simulink library "myLibrary"  (R2023b)
settings: Solver=VariableStepAuto  StartTime=0.0  StopTime=10.0  RelTol=1e-3
undefined symbols (not defined in the file): Cac_n1, ctrl1, Da, Discrete, dtha, ee_sli_rtmsupport, FA, gcbh, Ha, Ini, init_DCline, init_IPC, init_line, init_load, init_SG, init_shunt, init_TH, init_trafo, init_VSC, initMachineBlocks, Ka, Lf, Llkd_pu, Llkq1_pu, magnitude, NET, P, plots_step, q0, Rac_n1, Radd, Rkd_pu, Rkq1_pu, Rload_add, sim_config, sps_rtmsupport, spsSteamTurbineModel, T_DC_NET, T_global, T_IPC, T_load, T_NET, T_SG, T_shunt, T_STATCOM, T_TH, T_trafo, T_VSC, Ts, tstep, Udiff_a, V1
libraries: spsSeriesRLCBranchLib x105, eeGeneralControl x72, $bdroot x70, spsCurrentMeasurementLib x48, spsParallelRLCBranchLib x39, spsVoltageMeasurementLib x33, spsControlledVoltageSourceLib x27, spsFirstOrderFilterLib x16, dspsigops x6, spsThreePhaseVIMeasurementLib x5, spsPLL3phLib x4, spsThreePhaseBreakerLib x3
(part 7 of 12)

== system myLibrary/AC-GFOL_DC-GFOL/Control Pac2/PLL1 ==
  Ud : Inport
  Constant : Constant  Value=0
  Constant1 : Constant  Value=2*pi*T_IPC.fb
  Gain : Gain  Gain=T_IPC.kiPLL
  Gain1 : Gain  Gain=T_IPC.kpPLL
  Integrator : Integrator  InitialCondition=initIPC.thetaPLL_init
  Integrator1 : Integrator
  Scope : Scope
  Scope1 : Scope  NumInputPorts=2
  Sum : Sum  Inputs=|+-
  Sum1 : Sum  Inputs=|++
  Sum2 : Sum  Inputs=|++
  Angle : Outport
  w : Outport  Port=2
  wires:
  Ud/1 -> Scope1/2, Sum/2
  Constant1/1 -> Sum2/2
  Sum2/1 -> w/1, Scope/1, Integrator/1
  Sum1/1 -> Sum2/1
  Integrator1/1 -> Sum1/2
  Gain1/1 -> Sum1/1
  Gain/1 -> Integrator1/1
  Sum/1 -> Gain1/1, Gain/1
  Constant/1 -> Scope1/1, Sum/1
  Integrator/1 -> Angle/1

== system myLibrary/AC-GFOL_DC-GFOL/Control Pac2/Rotació ==
  V_q_diff : Inport
  V_d_diff : Inport  Port=2
  V_0_diff : Inport  Port=3
  Angle : Inport  Port=4
  Constant{2,5..7} (4 alike) : Constant  Value=0
  Constant8 : Constant
  Demux : Demux  Outputs=3
  Display : Display
  Gain1 : Gain  Gain=-1
  Matrix Concatenate : Concatenate  NumInputs=3  Mode=Multidimensional array  ConcatenateDimension=2
  Mux{,1..3} (4 alike) : Mux  Inputs=3
  Product : Product  Multiplication=Matrix(*)
  Trigonometric Function : Trigonometry  Operator=cos
  Trigonometric Function1 : Trigonometry
  Trigonometric Function2 : Trigonometry
  Trigonometric Function3 : Trigonometry  Operator=cos
  V_alfa_diff : Outport  VectorParamsAs1DForOutWhenUnconnected=off
  V_beta_diff : Outport  Port=2  VectorParamsAs1DForOutWhenUnconnected=off
  V_0 : Outport  Port=3  VectorParamsAs1DForOutWhenUnconnected=off
  wires:
  Trigonometric Function1/1 -> Gain1/1
  Constant2/1 -> Mux1/3
  Trigonometric Function3/1 -> Mux2/2
  Constant5/1 -> Mux2/3
  Constant6/1 -> Mux3/1
  Constant7/1 -> Mux3/2
  Constant8/1 -> Mux3/3
  Mux2/1 -> Matrix Concatenate/2
  Mux3/1 -> Matrix Concatenate/3
  Mux1/1 -> Matrix Concatenate/1
  Product/1 -> Demux/1
  Demux/1 -> V_alfa_diff/1
  Demux/2 -> V_beta_diff/1
  Demux/3 -> V_0/1
  Mux/1 -> Product/2
  Matrix Concatenate/1 -> Display/1, Product/1
  V_q_diff/1 -> Mux/1
  V_d_diff/1 -> Mux/2
  V_0_diff/1 -> Mux/3
  Trigonometric Function/1 -> Mux1/1
  Gain1/1 -> Mux1/2
  Trigonometric Function2/1 -> Mux2/1
  Angle/1 -> Trigonometric Function/1, Trigonometric Function3/1, Trigonometric Function2/1, Trigonometric Function1/1

== system myLibrary/AC-GFOL_DC-GFOL/Control Pac2/Subsystem ==
  iqs : Inport
  uq : Inport  Port=2
  ids : Inport  Port=3
  ud : Inport  Port=4
  w : Inport  Port=5
  Pac_ref : Inport  Port=6
  Constant : Constant  Value=T_IPC.fb*2*pi
  Display5 : Display
  Gain1 : Gain  Gain=T_IPC.kpw
  Gain2 : Gain  Gain=3/2
  Integrator1 : Integrator  InitialCondition=initIPC.idiffq
  Product3 : Product
  Product5 : Product
  Scope : Scope  NumInputPorts=2
  Scope1 : Scope
  Sum1 : Sum
  Sum10 : Sum  Inputs=|++
  Sum2 : Sum  Inputs=++-
  Sum3 : Sum  Inputs=|+-
  k7 : Gain  Gain=T_IPC.kiPac
  k8 : Gain  Gain=T_IPC.kpPac
  iqref : Outport
  wires:
  Constant/1 -> Sum3/1
  w/1 -> Sum3/2
  Sum3/1 -> Gain1/1
  Gain2/1 -> Sum2/3, Scope/2  "V_0_"
  iqs/1 -> Product3/2
  Product5/1 -> Sum1/2
  uq/1 -> Product3/1
  ids/1 -> Product5/2
  Sum1/1 -> Gain2/1  "V_0_s"
  ud/1 -> Product5/1
  Product3/1 -> Sum1/1
  Pac_ref/1 -> Scope/1, Sum2/2
  Integrator1/1 -> Display5/1, Scope1/1, Sum10/2
  k7/1 -> Integrator1/1
  k8/1 -> Sum10/1
  Sum2/1 -> k7/1, k8/1
  Sum10/1 -> iqref/1

== system myLibrary/AC-GFOL_DC-GFOL/Control Pac2/Subsystem1 ==
  uref : Inport
  uq : Inport  Port=2
  ud : Inport  Port=3
  Gain3 : Gain  Gain=T_IPC.kpVac
  Low-Pass Filter (Discrete or Continuous)2 : eeGeneralControl/Low-Pass Filter (Discrete or Continuous)  K=1  T=T_IPC.tVac  B=inf  A=-inf  init_option=Inherited from block input  x0=0  Ts=0
  Product4 : Product
  Product6 : Product
  Scope : Scope  NumInputPorts=2
  Sqrt : Sqrt
  Sum : Sum
  Sum3 : Sum  Inputs=|+-
  idref : Outport
  wires:
  uref/1 -> Scope/1, Sum3/1
  Product6/1 -> Sum/2
  Sqrt/1 -> Low-Pass Filter (Discrete or Continuous)2/1, Scope/2
  uq/1 -> Product4/2, Product4/1
  Sum/1 -> Sqrt/1
  ud/1 -> Product6/2, Product6/1
  Gain3/1 -> idref/1  "V_0_"
  Product4/1 -> Sum/1
  Low-Pass Filter (Discrete or Continuous)2/1 -> Sum3/2
  Sum3/1 -> Gain3/1

== system myLibrary/AC-GFOL_DC-GFOL/Control Pac2/Subsystem2 ==
  iqs : Inport
  uq : Inport  Port=2
  ids : Inport  Port=3
  ud : Inport  Port=4
  Pac_ref : Inport  Port=5
  Display5 : Display
  Gain2 : Gain  Gain=3/2
  Integrator1 : Integrator  InitialCondition=initIPC.idiffd
  Product3 : Product
  Product5 : Product
  Scope : Scope  NumInputPorts=2
  Scope1 : Scope
  Sum1 : Sum  Inputs=+-
  Sum10 : Sum  Inputs=|++
  Sum2 : Sum  Inputs=|+-
  k7 : Gain  Gain=T_IPC.kiQ
  k8 : Gain  Gain=T_IPC.kpQ
  iqref : Outport
  wires:
  Sum10/1 -> iqref/1
  Sum2/1 -> k8/1, k7/1
  k8/1 -> Sum10/1
  k7/1 -> Integrator1/1
  Integrator1/1 -> Scope1/1, Sum10/2, Display5/1
  Pac_ref/1 -> Sum2/1, Scope/1
  Product3/1 -> Sum1/1
  ud/1 -> Product5/1
  Sum1/1 -> Gain2/1  "V_0_s"
  uq/1 -> Product3/1
  Product5/1 -> Sum1/2
  Gain2/1 -> Sum2/2, Scope/2  "V_0_"
  ids/1 -> Product3/2
  iqs/1 -> Product5/2

== system myLibrary/AC-GFOL_DC-GFOL/Control Pac2/l_DC_alfa//beta ==
  Iabc_sum : Inport
  Clarke : Subsystem
  Ialfa_sum : Outport  VectorParamsAs1DForOutWhenUnconnected=off
  Ibeta_sum : Outport  Port=2  VectorParamsAs1DForOutWhenUnconnected=off
  I0_sum : Outport  Port=3  VectorParamsAs1DForOutWhenUnconnected=off
  wires:
  Clarke/1(I_alfa) -> Ialfa_sum/1
  Clarke/2(I_beta) -> Ibeta_sum/1
  Clarke/3(I_0) -> I0_sum/1
  Iabc_sum/1 -> Clarke/1(Isum)

== system myLibrary/AC-GFOL_DC-GFOR/Control Pac2/Calcul Energies2 ==
  Vs : Inport
  Demux : Demux  Outputs=6
  Gain{1..6} (6 alike) : Gain  Gain=T_IPC.Carm/2
  Math Function{1..6} (6 alike) : Math  Operator=magnitude^2  SignedPower=on
  Sum4 : Sum  Inputs=|++
  Sum5 : Sum  Inputs=|++
  Sum9 : Sum  Inputs=|++
  Eat : Outport
  Ebt : Outport  Port=2
  Ect : Outport  Port=3
  wires:
  [Ebl] -> Sum5/2
  Gain5/1 -> [Ecu]  "Ecu"
  [Eau] -> Sum4/1
  Gain1/1 -> [Eau]  "Eau"
  Gain2/1 -> [Eal]  "Eal"
  [Ecu] -> Sum9/1
  Math Function4/1 -> Gain4/1
  [Ecl] -> Sum9/2
  Math Function1/1 -> Gain1/1
  Gain4/1 -> [Ebl]  "Ebl"
  [Ebu] -> Sum5/1
  Gain6/1 -> [Ecl]  "Ecl"
  Sum9/1 -> Ect/1
  Math Function5/1 -> Gain5/1
  [Vcls] -> Math Function6/1
  Math Function2/1 -> Gain2/1
  [Vbus] -> Math Function3/1
  Sum5/1 -> Ebt/1
  Math Function6/1 -> Gain6/1
  [Vals] -> Math Function2/1
  [Vaus] -> Math Function1/1
  Math Function3/1 -> Gain3/1
  Sum4/1 -> Eat/1
  Gain3/1 -> [Ebu]  "Ebu"
  [Eal] -> Sum4/2
  [Vcus] -> Math Function5/1
  [Vbls] -> Math Function4/1
  Vs/1 -> Demux/1
  Demux/1 -> [Vaus]
  Demux/2 -> [Vals]
  Demux/3 -> [Vbus]
  Demux/4 -> [Vbls]
  Demux/5 -> [Vcus]
  Demux/6 -> [Vcls]

== system myLibrary/AC-GFOL_DC-GFOR/Control Pac2/Clarke Anti-Transformation ==
  V_alfa_diff : Inport
  V_beta_dfff : Inport  Port=2
  V_0_diff : Inport  Port=3
  Constant{,2,5,8} (4 alike) : Constant
  Constant1 : Constant  Value=0
  Constant3 : Constant  Value=-1/2
  Constant4 : Constant  Value=-sqrt(3)/2
  Constant6 : Constant  Value=-1/2
  Constant7 : Constant  Value=sqrt(3)/2
  Demux : Demux  Outputs=3
  Display : Display
  Math Function : Math  Operator=transpose  SignedPower=on
  Matrix Concatenate : Concatenate  NumInputs=3  Mode=Multidimensional array  ConcatenateDimension=2
  Mux{,1..3} (4 alike) : Mux  Inputs=3
  Product : Product  Multiplication=Matrix(*)
  Va_diff : Outport  VectorParamsAs1DForOutWhenUnconnected=off
  Vb_diff : Outport  Port=2  VectorParamsAs1DForOutWhenUnconnected=off
  Vc_diff : Outport  Port=3  VectorParamsAs1DForOutWhenUnconnected=off
  wires:
  Constant/1 -> Mux1/1
  Constant1/1 -> Mux1/2
  Constant2/1 -> Mux1/3
  Constant3/1 -> Mux2/1
  Constant4/1 -> Mux2/2
  Constant5/1 -> Mux2/3
  Constant6/1 -> Mux3/1
  Constant7/1 -> Mux3/2
  Constant8/1 -> Mux3/3
  Matrix Concatenate/1 -> Math Function/1
  Mux2/1 -> Matrix Concatenate/2
  Mux3/1 -> Matrix Concatenate/3
  Mux1/1 -> Matrix Concatenate/1
  Product/1 -> Demux/1
  Demux/1 -> Va_diff/1  "Va"
  Demux/2 -> Vb_diff/1  "Vb"
  Demux/3 -> Vc_diff/1  "Vc"
  Mux/1 -> Product/2
  Math Function/1 -> Display/1, Product/1
  V_alfa_diff/1 -> Mux/1  "Valfa"
  V_beta_dfff/1 -> Mux/2  "Vbeta"
  V_0_diff/1 -> Mux/3  "0"

== system myLibrary/AC-GFOL_DC-GFOR/Control Pac2/Clarke Anti-Transformation2 ==
  V_alfa_sum : Inport
  V_beta_sum : Inport  Port=2
  V_0_sum : Inport  Port=3
  Constant{,2,5,8} (4 alike) : Constant
  Constant1 : Constant  Value=0
  Constant3 : Constant  Value=-1/2
  Constant4 : Constant  Value=-sqrt(3)/2
  Constant6 : Constant  Value=-1/2
  Constant7 : Constant  Value=sqrt(3)/2
  Demux : Demux  Outputs=3
  Display : Display
  Math Function : Math  Operator=transpose  SignedPower=on
  Matrix Concatenate : Concatenate  NumInputs=3  Mode=Multidimensional array  ConcatenateDimension=2
  Mux{,1..3} (4 alike) : Mux  Inputs=3
  Product : Product  Multiplication=Matrix(*)
  Va_sum : Outport  VectorParamsAs1DForOutWhenUnconnected=off
  Vb_sum : Outport  Port=2  VectorParamsAs1DForOutWhenUnconnected=off
  Vc_sum : Outport  Port=3  VectorParamsAs1DForOutWhenUnconnected=off
  wires:
  Constant/1 -> Mux1/1
  Constant1/1 -> Mux1/2
  Constant2/1 -> Mux1/3
  Constant3/1 -> Mux2/1
  Constant4/1 -> Mux2/2
  Constant5/1 -> Mux2/3
  Constant6/1 -> Mux3/1
  Constant7/1 -> Mux3/2
  Constant8/1 -> Mux3/3
  Matrix Concatenate/1 -> Math Function/1
  Mux2/1 -> Matrix Concatenate/2
  Mux3/1 -> Matrix Concatenate/3
  Mux1/1 -> Matrix Concatenate/1
  Product/1 -> Demux/1
  Demux/1 -> Va_sum/1  "Va"
  Demux/2 -> Vb_sum/1  "Vb"
  Demux/3 -> Vc_sum/1  "Vc"
  Mux/1 -> Product/2
  Math Function/1 -> Display/1, Product/1
  V_alfa_sum/1 -> Mux/1  "Valfa"
  V_beta_sum/1 -> Mux/2  "Vbeta"
  V_0_sum/1 -> Mux/3  "0"

== system myLibrary/AC-GFOL_DC-GFOR/Control Pac2/Conditional zoh1 ==
  In1 : Inport
  Constant4 : Constant  Value=T_IPC.tau_zoh
  Switch : Switch  Criteria=u2 > Threshold  SaturateOnIntegerOverflow=off  InputSameDT=off
  Zero-Order Hold9 : ZeroOrderHold  SampleTime=T_IPC.tau_zoh
  Out1 : Outport
  wires:
  In1/1 -> Zero-Order Hold9/1, Switch/3
  Zero-Order Hold9/1 -> Switch/1
  Constant4/1 -> Switch/2
  Switch/1 -> Out1/1

== system myLibrary/AC-GFOL_DC-GFOR/Control Pac2/Conditional zoh5 ==
  In1 : Inport
  Constant4 : Constant  Value=T_IPC.tau_zoh
  Switch : Switch  Criteria=u2 > Threshold  SaturateOnIntegerOverflow=off  InputSameDT=off
  Zero-Order Hold9 : ZeroOrderHold  SampleTime=T_IPC.tau_zoh
  Out1 : Outport
  wires:
  In1/1 -> Zero-Order Hold9/1, Switch/3
  Zero-Order Hold9/1 -> Switch/1
  Constant4/1 -> Switch/2
  Switch/1 -> Out1/1

== system myLibrary/AC-GFOL_DC-GFOR/Control Pac2/Conditional zoh7 ==
  In1 : Inport
  Constant4 : Constant  Value=T_IPC.tau_zoh
  Switch : Switch  Criteria=u2 > Threshold  SaturateOnIntegerOverflow=off  InputSameDT=off
  Zero-Order Hold9 : ZeroOrderHold  SampleTime=T_IPC.tau_zoh
  Out1 : Outport
  wires:
  Switch/1 -> Out1/1
  Constant4/1 -> Switch/2
  Zero-Order Hold9/1 -> Switch/1
  In1/1 -> Switch/3, Zero-Order Hold9/1

== system myLibrary/AC-GFOL_DC-GFOR/Control Pac2/Conditional zoh8 ==
  In1 : Inport
  Constant4 : Constant  Value=T_IPC.tau_zoh
  Switch : Switch  Criteria=u2 > Threshold  SaturateOnIntegerOverflow=off  InputSameDT=off
  Zero-Order Hold9 : ZeroOrderHold  SampleTime=T_IPC.tau_zoh
  Out1 : Outport
  wires:
  Switch/1 -> Out1/1
  Constant4/1 -> Switch/2
  Zero-Order Hold9/1 -> Switch/1
  In1/1 -> Switch/3, Zero-Order Hold9/1

== system myLibrary/AC-GFOL_DC-GFOR/Control Pac2/Control Energies DC ==
  Pt : Inport
  Display1 : Display
  Integrator1 : Integrator  InitialCondition=initIPC.PI_Wt
  Scope : Scope
  Sum10 : Sum  Inputs=|++
  k7 : Gain  Gain=T_IPC.kiEt
  k8 : Gain  Gain=T_IPC.kpEt
  Pt' : Outport  VectorParamsAs1DForOutWhenUnconnected=off
  wires:
  Sum10/1 -> Pt'/1  "Pt"
  k7/1 -> Integrator1/1
  Pt/1 -> k7/1, k8/1
  k8/1 -> Sum10/1
  Integrator1/1 -> Scope/1, Sum10/2, Display1/1

== system myLibrary/AC-GFOL_DC-GFOR/Control Pac2/Controladors ==
  I_0_sum : Inport
  Display : Display
  Gain2 : Gain  Gain=-1
  Integrator1 : Integrator  InitialCondition=initIPC.PI_isum0_DC
  Ki1 : Gain  Gain=T_IPC.kiIsum
  Kp1 : Gain  Gain=T_IPC.kpIsum
  Scope : Scope
  Sum5 : Sum
  V_0_sum : Outport  VectorParamsAs1DForOutWhenUnconnected=off
  wires:
  Sum5/1 -> Gain2/1
  Gain2/1 -> V_0_sum/1
  Ki1/1 -> Integrator1/1
  Integrator1/1 -> Display/1, Scope/1, Sum5/1
  Kp1/1 -> Sum5/2
  I_0_sum/1 -> Kp1/1, Ki1/1

== system myLibrary/AC-GFOL_DC-GFOR/Control Pac2/Current Control ==
  Iq* : Inport
  Iq : Inport  Port=2
  Id* : Inport  Port=3
  Id : Inport  Port=4
  uq : Inport  Port=5
  ud : Inport  Port=6
  Constant : Constant  Value=2*pi*T_IPC.fb
  Display1 : Display
  Display6 : Display
  Id1 : InportShadow  Port=4
  Integrator : Integrator  InitialCondition=initIPC.PI_idiffq
  Integrator1 : Integrator  InitialCondition=initIPC.PI_idiffd
  Iq1 : InportShadow  Port=2
  Ki : Gain  Gain=T_IPC.kiIs
  Ki1 : Gain  Gain=T_IPC.kiIs
  Kp : Gain  Gain=T_IPC.kpIs
  Kp1 : Gain  Gain=T_IPC.kpIs
  Kp2 : Gain  Gain=T_IPC.Lc+T_IPC.La/2
  Product : Product
  Product1 : Product
  Scope : Scope  NumInputPorts=2
  Scope1 : Scope  NumInputPorts=2
  Sum : Sum  Inputs=|+-
  Sum1 : Sum  Inputs=|+-
  Sum2 : Sum  Inputs=+++
  Sum3 : Sum  Inputs=-++
  Sum4 : Sum
  Sum5 : Sum
  V_q_s : Outport  VectorParamsAs1DForOutWhenUnconnected=off
  V_d_s : Outport  Port=2  VectorParamsAs1DForOutWhenUnconnected=off
  wires:
  Sum2/1 -> V_q_s/1
  Sum5/1 -> Sum3/2
  Kp1/1 -> Sum5/2
  Integrator1/1 -> Display1/1, Sum5/1
  Ki1/1 -> Integrator1/1
  Sum1/1 -> Ki1/1, Kp1/1  "Error"
  Kp/1 -> Sum4/2
  Integrator/1 -> Display6/1, Sum4/1
  Ki/1 -> Integrator/1
  Sum/1 -> Kp/1, Ki/1
  Id*/1 -> Scope1/1, Sum1/1
  Kp2/1 -> Product/2, Product1/1
  Id/1 -> Scope1/2, Sum1/2
  Iq/1 -> Scope/2, Sum/2
  Iq*/1 -> Scope/1, Sum/1
  Constant/1 -> Kp2/1
  ud/1 -> Sum3/3
  Sum4/1 -> Sum2/1
  uq/1 -> Sum2/3
  Sum3/1 -> V_d_s/1
  Product/1 -> Sum3/1
  Product1/1 -> Sum2/2
  Iq1/1 -> Product/1
  Id1/1 -> Product1/2

== system myLibrary/AC-GFOL_DC-GFOR/Control Pac2/Is ==
  Ias : Inport
  Ibs : Inport  Port=2
  Ics : Inport  Port=3
  Angle : Inport  Port=4
  Demux1 : Demux  Outputs=3
  Matriu T : Subsystem
  Mux : Mux  Inputs=3
  Product : Product  Multiplication=Matrix(*)
  I_q_s : Outport  VectorParamsAs1DForOutWhenUnconnected=off
  I_d_s : Outport  Port=2  VectorParamsAs1DForOutWhenUnconnected=off
  I_0_s : Outport  Port=3  VectorParamsAs1DForOutWhenUnconnected=off
  wires:
  Product/1 -> Demux1/1
  Matriu T/1(Out1) -> Product/1
  Demux1/1 -> I_q_s/1
  Demux1/2 -> I_d_s/1
  Demux1/3 -> I_0_s/1
  Angle/1 -> Matriu T/1(u)
  Mux/1 -> Product/2
  Ias/1 -> Mux/1
  Ibs/1 -> Mux/2
  Ics/1 -> Mux/3

== system myLibrary/AC-GFOL_DC-GFOR/Control Pac2/Is2 ==
  Ias : Inport
  Ibs : Inport  Port=2
  Ics : Inport  Port=3
  Angle : Inport  Port=4
  Demux1 : Demux  Outputs=3
  Matriu T : Subsystem
  Mux : Mux  Inputs=3
  Product : Product  Multiplication=Matrix(*)
  I_q_s : Outport  VectorParamsAs1DForOutWhenUnconnected=off
  I_d_s : Outport  Port=2  VectorParamsAs1DForOutWhenUnconnected=off
  I_0_s : Outport  Port=3  VectorParamsAs1DForOutWhenUnconnected=off
  wires:
  Product/1 -> Demux1/1
  Matriu T/1(Out1) -> Product/1
  Demux1/1 -> I_q_s/1
  Demux1/2 -> I_d_s/1
  Demux1/3 -> I_0_s/1
  Angle/1 -> Matriu T/1(u)
  Mux/1 -> Product/2
  Ias/1 -> Mux/1
  Ibs/1 -> Mux/2
  Ics/1 -> Mux/3

== system myLibrary/AC-GFOL_DC-GFOR/Control Pac2/PLL1 ==
  Ud : Inport
  Constant : Constant  Value=0
  Constant1 : Constant  Value=2*pi*T_IPC.fb
  Gain : Gain  Gain=T_IPC.kiPLL
  Gain1 : Gain  Gain=T_IPC.kpPLL
  Integrator : Integrator  InitialCondition=initIPC.thetaPLL_init
  Integrator1 : Integrator
  Scope : Scope
  Scope1 : Scope  NumInputPorts=2
  Sum : Sum  Inputs=|+-
  Sum1 : Sum  Inputs=|++
  Sum2 : Sum  Inputs=|++
  Angle : Outport
  w : Outport  Port=2
  wires:
  Ud/1 -> Scope1/2, Sum/2
  Constant1/1 -> Sum2/2
  Sum2/1 -> w/1, Scope/1, Integrator/1
  Sum1/1 -> Sum2/1
  Integrator1/1 -> Sum1/2
  Gain1/1 -> Sum1/1
  Gain/1 -> Integrator1/1
  Sum/1 -> Gain1/1, Gain/1
  Constant/1 -> Scope1/1, Sum/1
  Integrator/1 -> Angle/1

== system myLibrary/AC-GFOL_DC-GFOR/Control Pac2/Rotació ==
  V_q_diff : Inport
  V_d_diff : Inport  Port=2
  V_0_diff : Inport  Port=3
  Angle : Inport  Port=4
  Constant{2,5..7} (4 alike) : Constant  Value=0
  Constant8 : Constant
  Demux : Demux  Outputs=3
  Display : Display
  Gain1 : Gain  Gain=-1
  Matrix Concatenate : Concatenate  NumInputs=3  Mode=Multidimensional array  ConcatenateDimension=2
  Mux{,1..3} (4 alike) : Mux  Inputs=3
  Product : Product  Multiplication=Matrix(*)
  Trigonometric Function : Trigonometry  Operator=cos
  Trigonometric Function1 : Trigonometry
  Trigonometric Function2 : Trigonometry
  Trigonometric Function3 : Trigonometry  Operator=cos
  V_alfa_diff : Outport  VectorParamsAs1DForOutWhenUnconnected=off
  V_beta_diff : Outport  Port=2  VectorParamsAs1DForOutWhenUnconnected=off
  V_0 : Outport  Port=3  VectorParamsAs1DForOutWhenUnconnected=off
  wires:
  Trigonometric Function1/1 -> Gain1/1
  Constant2/1 -> Mux1/3
  Trigonometric Function3/1 -> Mux2/2
  Constant5/1 -> Mux2/3
  Constant6/1 -> Mux3/1
  Constant7/1 -> Mux3/2
  Constant8/1 -> Mux3/3
  Mux2/1 -> Matrix Concatenate/2
  Mux3/1 -> Matrix Concatenate/3
  Mux1/1 -> Matrix Concatenate/1
  Product/1 -> Demux/1
  Demux/1 -> V_alfa_diff/1
  Demux/2 -> V_beta_diff/1
  Demux/3 -> V_0/1
  Mux/1 -> Product/2
  Matrix Concatenate/1 -> Display/1, Product/1
  V_q_diff/1 -> Mux/1
  V_d_diff/1 -> Mux/2
  V_0_diff/1 -> Mux/3
  Trigonometric Function/1 -> Mux1/1
  Gain1/1 -> Mux1/2
  Trigonometric Function2/1 -> Mux2/1
  Angle/1 -> Trigonometric Function/1, Trigonometric Function3/1, Trigonometric Function2/1, Trigonometric Function1/1

== system myLibrary/AC-GFOL_DC-GFOR/Control Pac2/Subsystem1 ==
  uref : Inport
  uq : Inport  Port=2
  ud : Inport  Port=3
  Gain3 : Gain  Gain=T_IPC.kpVac
  Low-Pass Filter (Discrete or Continuous)2 : eeGeneralControl/Low-Pass Filter (Discrete or Continuous)  K=1  T=T_IPC.tVac  B=inf  A=-inf  init_option=Inherited from block input  x0=0  Ts=0
  Product4 : Product
  Product6 : Product
  Scope : Scope  NumInputPorts=2
  Sqrt : Sqrt
  Sum : Sum
  Sum3 : Sum  Inputs=|+-
  idref : Outport
  wires:
  uref/1 -> Scope/1, Sum3/1
  Product6/1 -> Sum/2
  Sqrt/1 -> Low-Pass Filter (Discrete or Continuous)2/1, Scope/2
  uq/1 -> Product4/2, Product4/1
  Sum/1 -> Sqrt/1
  ud/1 -> Product6/2, Product6/1
  Gain3/1 -> idref/1  "V_0_"
  Product4/1 -> Sum/1
  Low-Pass Filter (Discrete or Continuous)2/1 -> Sum3/2
  Sum3/1 -> Gain3/1

== system myLibrary/AC-GFOL_DC-GFOR/Control Pac2/Subsystem2 ==
  iqs : Inport
  uq : Inport  Port=2
  ids : Inport  Port=3
  ud : Inport  Port=4
  w : Inport  Port=5
  Vdc_ref : Inport  Port=6
  Pac_ref : Inport  Port=7
  Vdc : Inport  Port=8
  Constant : Constant  Value=T_IPC.fb*2*pi
  Display : Display
  Display5 : Display
  Gain1 : Gain  Gain=T_IPC.kpw
  Gain2 : Gain  Gain=3/2
  Gain3 : Gain  Gain=T_IPC.kpVdc
  Gain4 : Gain  Commented=on  Gain=T_IPC.kiVdc
  Integrator1 : Integrator  InitialCondition=initIPC.idiffq
  Integrator2 : Integrator  Commented=on
  Product3 : Product
  Product5 : Product
  Scope : Scope  NumInputPorts=2
  Scope1 : Scope
  Scope2 : Scope
  Sum : Sum  Inputs=|+-
  Sum1 : Sum
  Sum10 : Sum  Inputs=|++
  Sum2 : Sum  Inputs=++-+
  Sum3 : Sum  Inputs=|+-
  Sum4 : Sum  Inputs=|++
  k1 : Gain  Gain=-1
  k7 : Gain  Gain=T_IPC.kiPac
  k8 : Gain  Gain=T_IPC.kpPac
  iqref : Outport
  wires:
  Sum/1 -> Gain4/1, Gain3/1
  Integrator1/1 -> Display5/1, Sum10/2
  k7/1 -> Integrator1/1
  k8/1 -> Sum10/1
  Vdc/1 -> Sum/2, Scope/2
  Vdc_ref/1 -> Sum/1, Scope/1
  Product3/1 -> Sum1/1
  ud/1 -> Product5/1
  ids/1 -> Product5/2
  Sum10/1 -> iqref/1
  uq/1 -> Product3/1
  Product5/1 -> Sum1/2
  Sum2/1 -> k8/1, k7/1
  iqs/1 -> Product3/2
  Sum1/1 -> Gain2/1
  Sum3/1 -> Gain1/1
  Constant/1 -> Sum3/1
  w/1 -> Sum3/2
  Pac_ref/1 -> Sum2/2
  Gain2/1 -> Display/1, Scope1/1, Sum2/3  "Pac"
  Gain3/1 -> Sum4/1  "Pac"
  Gain4/1 -> Integrator2/1  "Pac"
  Integrator2/1 -> Sum4/2
  Sum4/1 -> k1/1
  k1/1 -> Sum2/1

== system myLibrary/AC-GFOL_DC-GFOR/Control Pac2/Subsystem3 ==
  iqs : Inport
  uq : Inport  Port=2
  ids : Inport  Port=3
  ud : Inport  Port=4
  Pac_ref : Inport  Port=5
  Display : Display
  Display5 : Display
  Gain2 : Gain  Gain=3/2
  Integrator1 : Integrator  InitialCondition=initIPC.idiffd
  Product3 : Product
  Product5 : Product
  Scope1 : Scope  NumInputPorts=2
  Sum1 : Sum  Inputs=+-
  Sum10 : Sum  Inputs=|++
  Sum2 : Sum  Inputs=|+-
  k7 : Gain  Gain=T_IPC.kiQ
  k8 : Gain  Gain=T_IPC.kpQ
  iqref : Outport
  wires:
  Integrator1/1 -> Display5/1, Sum10/2
  k7/1 -> Integrator1/1
  k8/1 -> Sum10/1
  Product3/1 -> Sum1/1
  ud/1 -> Product5/1
  Sum10/1 -> iqref/1
  uq/1 -> Product3/1
  Product5/1 -> Sum1/2
  Sum2/1 -> k8/1, k7/1
  Sum1/1 -> Gain2/1
  Gain2/1 -> Sum2/2, Display/1, Scope1/2  "Pac"
  Pac_ref/1 -> Scope1/1, Sum2/1
  ids/1 -> Product3/2
  iqs/1 -> Product5/2

== system myLibrary/AC-GFOL_DC-GFOR/Control Pac2/l_DC_alfa//beta ==
  Iabc_sum : Inport
  Clarke : Subsystem
  Ialfa_sum : Outport  VectorParamsAs1DForOutWhenUnconnected=off
  Ibeta_sum : Outport  Port=2  VectorParamsAs1DForOutWhenUnconnected=off
  I0_sum : Outport  Port=3  VectorParamsAs1DForOutWhenUnconnected=off
  wires:
  Clarke/1(I_alfa) -> Ialfa_sum/1
  Clarke/2(I_beta) -> Ibeta_sum/1
  Clarke/3(I_0) -> I0_sum/1
  Iabc_sum/1 -> Clarke/1(Isum)

== system myLibrary/AC-GFOL_DC-GFOR/MMC1/Controlled Voltage Source2 ==
  s : Inport
  ControlledVoltageSource : PMComponent  PhysicalDomain=powersysdomain  LeftPortType=p1  RightPortType=p1  LConnTagsString=a  RConnTagsString=__new0  mask(InnerPowersysBlock){}
      mask Display: disp('SPS internal use\nDo not delete')
  - : PMIOPort  Side=Left
  + : PMIOPort  Port=2  Side=Right
  tag scope: LibraryTag=global
  wires:
  s/1 -> [LibraryTag]
  connections:
  -/RConn1 -- ControlledVoltageSource/LConn1
  ControlledVoltageSource/RConn1 -- +/RConn1

== system myLibrary/AC-GFOL_DC-GFOR/MMC1/Controlled Voltage Source3 ==
  s : Inport
  ControlledVoltageSource : PMComponent  PhysicalDomain=powersysdomain  LeftPortType=p1  RightPortType=p1  LConnTagsString=a  RConnTagsString=__new0  mask(InnerPowersysBlock){}
      mask Display: disp('SPS internal use\nDo not delete')
  - : PMIOPort  Side=Left
  + : PMIOPort  Port=2  Side=Right
  tag scope: LibraryTag=global
  wires:
  s/1 -> [LibraryTag]
  connections:
  ControlledVoltageSource/RConn1 -- +/RConn1
  -/RConn1 -- ControlledVoltageSource/LConn1

== system myLibrary/AC-GFOR_DC-GFOL/Control Pac2/Calcul Energies2 ==
  Vs : Inport
  Demux : Demux  Outputs=6
  Gain{1..6} (6 alike) : Gain  Gain=T_IPC.Carm/2
  Math Function{1..6} (6 alike) : Math  Operator=magnitude^2  SignedPower=on
  Sum4 : Sum  Inputs=|++
  Sum5 : Sum  Inputs=|++
  Sum9 : Sum  Inputs=|++
  Eat : Outport
  Ebt : Outport  Port=2
  Ect : Outport  Port=3
  wires:
  Demux/6 -> [Vcls]
  Demux/5 -> [Vcus]
  Demux/4 -> [Vbls]
  Demux/3 -> [Vbus]
  Demux/2 -> [Vals]
  Demux/1 -> [Vaus]
  Vs/1 -> Demux/1
  [Vbls] -> Math Function4/1
  [Vcus] -> Math Function5/1
  [Eal] -> Sum4/2
  Gain3/1 -> [Ebu]  "Ebu"
  Sum4/1 -> Eat/1
  Math Function3/1 -> Gain3/1
  [Vaus] -> Math Function1/1
  [Vals] -> Math Function2/1
  Math Function6/1 -> Gain6/1
  Sum5/1 -> Ebt/1
  [Vbus] -> Math Function3/1
  Math Function2/1 -> Gain2/1
  [Vcls] -> Math Function6/1
  Math Function5/1 -> Gain5/1
  Sum9/1 -> Ect/1
  Gain6/1 -> [Ecl]  "Ecl"
  [Ebu] -> Sum5/1
  Gain4/1 -> [Ebl]  "Ebl"
  Math Function1/1 -> Gain1/1
  [Ecl] -> Sum9/2
  Math Function4/1 -> Gain4/1
  [Ecu] -> Sum9/1
  Gain2/1 -> [Eal]  "Eal"
  Gain1/1 -> [Eau]  "Eau"
  [Eau] -> Sum4/1
  Gain5/1 -> [Ecu]  "Ecu"
  [Ebl] -> Sum5/2

== system myLibrary/AC-GFOR_DC-GFOL/Control Pac2/Clarke Anti-Transformation ==
  V_alfa_diff : Inport
  V_beta_dfff : Inport  Port=2
  V_0_diff : Inport  Port=3
  Constant{,2,5,8} (4 alike) : Constant
  Constant1 : Constant  Value=0
  Constant3 : Constant  Value=-1/2
  Constant4 : Constant  Value=-sqrt(3)/2
  Constant6 : Constant  Value=-1/2
  Constant7 : Constant  Value=sqrt(3)/2
  Demux : Demux  Outputs=3
  Display : Display
  Math Function : Math  Operator=transpose  SignedPower=on
  Matrix Concatenate : Concatenate  NumInputs=3  Mode=Multidimensional array  ConcatenateDimension=2
  Mux{,1..3} (4 alike) : Mux  Inputs=3
  Product : Product  Multiplication=Matrix(*)
  Va_diff : Outport  VectorParamsAs1DForOutWhenUnconnected=off
  Vb_diff : Outport  Port=2  VectorParamsAs1DForOutWhenUnconnected=off
  Vc_diff : Outport  Port=3  VectorParamsAs1DForOutWhenUnconnected=off
  wires:
  V_0_diff/1 -> Mux/3  "0"
  V_beta_dfff/1 -> Mux/2  "Vbeta"
  V_alfa_diff/1 -> Mux/1  "Valfa"
  Math Function/1 -> Product/1, Display/1
  Mux/1 -> Product/2
  Demux/3 -> Vc_diff/1  "Vc"
  Demux/2 -> Vb_diff/1  "Vb"
  Demux/1 -> Va_diff/1  "Va"
  Product/1 -> Demux/1
  Mux1/1 -> Matrix Concatenate/1
  Mux3/1 -> Matrix Concatenate/3
  Mux2/1 -> Matrix Concatenate/2
  Matrix Concatenate/1 -> Math Function/1
  Constant8/1 -> Mux3/3
  Constant7/1 -> Mux3/2
  Constant6/1 -> Mux3/1
  Constant5/1 -> Mux2/3
  Constant4/1 -> Mux2/2
  Constant3/1 -> Mux2/1
  Constant2/1 -> Mux1/3
  Constant1/1 -> Mux1/2
  Constant/1 -> Mux1/1

== system myLibrary/AC-GFOR_DC-GFOL/Control Pac2/Clarke Anti-Transformation2 ==
  V_alfa_sum : Inport
  V_beta_sum : Inport  Port=2
  V_0_sum : Inport  Port=3
  Constant{,2,5,8} (4 alike) : Constant
  Constant1 : Constant  Value=0
  Constant3 : Constant  Value=-1/2
  Constant4 : Constant  Value=-sqrt(3)/2
  Constant6 : Constant  Value=-1/2
  Constant7 : Constant  Value=sqrt(3)/2
  Demux : Demux  Outputs=3
  Display : Display
  Math Function : Math  Operator=transpose  SignedPower=on
  Matrix Concatenate : Concatenate  NumInputs=3  Mode=Multidimensional array  ConcatenateDimension=2
  Mux{,1..3} (4 alike) : Mux  Inputs=3
  Product : Product  Multiplication=Matrix(*)
  Va_sum : Outport  VectorParamsAs1DForOutWhenUnconnected=off
  Vb_sum : Outport  Port=2  VectorParamsAs1DForOutWhenUnconnected=off
  Vc_sum : Outport  Port=3  VectorParamsAs1DForOutWhenUnconnected=off
  wires:
  V_0_sum/1 -> Mux/3  "0"
  V_beta_sum/1 -> Mux/2  "Vbeta"
  V_alfa_sum/1 -> Mux/1  "Valfa"
  Math Function/1 -> Product/1, Display/1
  Mux/1 -> Product/2
  Demux/3 -> Vc_sum/1  "Vc"
  Demux/2 -> Vb_sum/1  "Vb"
  Demux/1 -> Va_sum/1  "Va"
  Product/1 -> Demux/1
  Mux1/1 -> Matrix Concatenate/1
  Mux3/1 -> Matrix Concatenate/3
  Mux2/1 -> Matrix Concatenate/2
  Matrix Concatenate/1 -> Math Function/1
  Constant8/1 -> Mux3/3
  Constant7/1 -> Mux3/2
  Constant6/1 -> Mux3/1
  Constant5/1 -> Mux2/3
  Constant4/1 -> Mux2/2
  Constant3/1 -> Mux2/1
  Constant2/1 -> Mux1/3
  Constant1/1 -> Mux1/2
  Constant/1 -> Mux1/1

== system myLibrary/AC-GFOR_DC-GFOL/Control Pac2/Conditional zoh1 ==
  In1 : Inport
  Constant4 : Constant  Value=T_IPC.tau_zoh
  Switch : Switch  Criteria=u2 > Threshold  SaturateOnIntegerOverflow=off  InputSameDT=off
  Zero-Order Hold9 : ZeroOrderHold  SampleTime=T_IPC.tau_zoh
  Out1 : Outport
  wires:
  In1/1 -> Zero-Order Hold9/1, Switch/3
  Zero-Order Hold9/1 -> Switch/1
  Constant4/1 -> Switch/2
  Switch/1 -> Out1/1

== system myLibrary/AC-GFOR_DC-GFOL/Control Pac2/Conditional zoh6 ==
  In1 : Inport
  Constant4 : Constant  Value=T_IPC.tau_zoh
  Switch : Switch  Criteria=u2 > Threshold  SaturateOnIntegerOverflow=off  InputSameDT=off
  Zero-Order Hold9 : ZeroOrderHold  SampleTime=T_IPC.tau_zoh
  Out1 : Outport
  wires:
  In1/1 -> Zero-Order Hold9/1, Switch/3
  Zero-Order Hold9/1 -> Switch/1
  Constant4/1 -> Switch/2
  Switch/1 -> Out1/1

== system myLibrary/AC-GFOR_DC-GFOL/Control Pac2/Control Energies DC ==
  Pt : Inport
  Display1 : Display
  Integrator1 : Integrator  InitialCondition=initIPC.PI_Wt
  Sum10 : Sum  Inputs=|++
  k7 : Gain  Gain=T_IPC.kiEt
  k8 : Gain  Gain=T_IPC.kpEt
  Pt' : Outport  VectorParamsAs1DForOutWhenUnconnected=off
  wires:
  k8/1 -> Sum10/1
  Pt/1 -> k8/1, k7/1
  k7/1 -> Integrator1/1
  Integrator1/1 -> Display1/1, Sum10/2
  Sum10/1 -> Pt'/1  "Pt"

== system myLibrary/AC-GFOR_DC-GFOL/Control Pac2/Controladors ==
  I_0_sum : Inport
  Gain2 : Gain  Gain=-1
  Integrator1 : Integrator  InitialCondition=initIPC.PI_isum0_DC
  Ki1 : Gain  Gain=T_IPC.kiIsum
  Kp1 : Gain  Gain=T_IPC.kpIsum
  Sum5 : Sum
  V_0_sum : Outport  VectorParamsAs1DForOutWhenUnconnected=off
  wires:
  I_0_sum/1 -> Ki1/1, Kp1/1
  Kp1/1 -> Sum5/2
  Integrator1/1 -> Sum5/1
  Ki1/1 -> Integrator1/1
  Gain2/1 -> V_0_sum/1
  Sum5/1 -> Gain2/1

== system myLibrary/AC-GFOR_DC-GFOL/Control Pac2/Current Control ==
  Iq* : Inport
  Iq : Inport  Port=2
  Id* : Inport  Port=3
  Id : Inport  Port=4
  uq : Inport  Port=5
  ud : Inport  Port=6
  Constant : Constant  Value=2*pi*T_IPC.fb
  Display1 : Display
  Display6 : Display
  Id1 : InportShadow  Port=4
  Integrator : Integrator  InitialCondition=initIPC.PI_idiffq
  Integrator1 : Integrator  InitialCondition=initIPC.PI_idiffd
  Iq1 : InportShadow  Port=2
  Ki : Gain  Gain=T_IPC.kiIs
  Ki1 : Gain  Gain=T_IPC.kiIs
  Kp : Gain  Gain=T_IPC.kpIs
  Kp1 : Gain  Gain=T_IPC.kpIs
  Kp2 : Gain  Gain=T_IPC.Lc+T_IPC.La/2
  Product : Product
  Product1 : Product
  Scope : Scope  NumInputPorts=2
  Scope1 : Scope  NumInputPorts=2
  Sum : Sum  Inputs=|+-
  Sum1 : Sum  Inputs=|+-
  Sum2 : Sum  Inputs=+++
  Sum3 : Sum  Inputs=-++
  Sum4 : Sum
  Sum5 : Sum
  V_q_s : Outport  VectorParamsAs1DForOutWhenUnconnected=off
  V_d_s : Outport  Port=2  VectorParamsAs1DForOutWhenUnconnected=off
  wires:
  Id1/1 -> Product1/2
  Iq1/1 -> Product/1
  Product1/1 -> Sum2/2
  Product/1 -> Sum3/1
  Sum3/1 -> V_d_s/1
  uq/1 -> Sum2/3
  Sum4/1 -> Sum2/1
  ud/1 -> Sum3/3
  Constant/1 -> Kp2/1
  Iq*/1 -> Sum/1, Scope/1
  Iq/1 -> Sum/2, Scope/2
  Id/1 -> Sum1/2, Scope1/2
  Kp2/1 -> Product1/1, Product/2
  Id*/1 -> Sum1/1, Scope1/1
  Sum/1 -> Ki/1, Kp/1
  Ki/1 -> Integrator/1
  Integrator/1 -> Sum4/1, Display6/1
  Kp/1 -> Sum4/2
  Sum1/1 -> Kp1/1, Ki1/1  "Error"
  Ki1/1 -> Integrator1/1
  Integrator1/1 -> Sum5/1, Display1/1
  Kp1/1 -> Sum5/2
  Sum5/1 -> Sum3/2
  Sum2/1 -> V_q_s/1

== system myLibrary/AC-GFOR_DC-GFOL/Control Pac2/Is ==
  Ias : Inport
  Ibs : Inport  Port=2
  Ics : Inport  Port=3
  Angle : Inport  Port=4
  Demux1 : Demux  Outputs=3
  Matriu T : Subsystem
  Mux : Mux  Inputs=3
  Product : Product  Multiplication=Matrix(*)
  I_q_s : Outport  VectorParamsAs1DForOutWhenUnconnected=off
  I_d_s : Outport  Port=2  VectorParamsAs1DForOutWhenUnconnected=off
  I_0_s : Outport  Port=3  VectorParamsAs1DForOutWhenUnconnected=off
  wires:
  Ics/1 -> Mux/3
  Ibs/1 -> Mux/2
  Ias/1 -> Mux/1
  Mux/1 -> Product/2
  Angle/1 -> Matriu T/1(u)
  Demux1/3 -> I_0_s/1
  Demux1/2 -> I_d_s/1
  Demux1/1 -> I_q_s/1
  Matriu T/1(Out1) -> Product/1
  Product/1 -> Demux1/1

== system myLibrary/AC-GFOR_DC-GFOL/Control Pac2/Is2 ==
  Ias : Inport
  Ibs : Inport  Port=2
  Ics : Inport  Port=3
  Angle : Inport  Port=4
  Demux1 : Demux  Outputs=3
  Matriu T : Subsystem
  Mux : Mux  Inputs=3
  Product : Product  Multiplication=Matrix(*)
  I_q_s : Outport  VectorParamsAs1DForOutWhenUnconnected=off
  I_d_s : Outport  Port=2  VectorParamsAs1DForOutWhenUnconnected=off
  I_0_s : Outport  Port=3  VectorParamsAs1DForOutWhenUnconnected=off
  wires:
  Ics/1 -> Mux/3
  Ibs/1 -> Mux/2
  Ias/1 -> Mux/1
  Mux/1 -> Product/2
  Angle/1 -> Matriu T/1(u)
  Demux1/3 -> I_0_s/1
  Demux1/2 -> I_d_s/1
  Demux1/1 -> I_q_s/1
  Matriu T/1(Out1) -> Product/1
  Product/1 -> Demux1/1

== system myLibrary/AC-GFOR_DC-GFOL/Control Pac2/PLL1 ==
  Pref : Inport
  iqs : Inport  Port=2
  uq : Inport  Port=3
  ids : Inport  Port=4
  ud : Inport  Port=5
  Constant4 : Constant  Value=2*pi*T_IPC.fb
  Gain5 : Gain  Gain=3/2
  Integrator2 : Integrator  InitialCondition=initIPC.thetaPLL_init
  Low-Pass Filter (Discrete or Continuous)2 : eeGeneralControl/Low-Pass Filter (Discrete or Continuous)  K=1  T=T_IPC.tPac  B=inf  A=-inf  init_option=Inherited from block input  x0=0  Ts=0
  Product3 : Product
  Product5 : Product
  Scope4 : Scope
  Sum18 : Sum  Inputs=++|
  Sum3 : Sum
  Sum35 : Sum  Inputs=|+-
  kdroop : Gain  Gain=T_IPC.kf
  Angle : Outport
  wires:
  ud/1 -> Product5/1
  uq/1 -> Product3/1
  Integrator2/1 -> Angle/1
  kdroop/1 -> Sum18/2
  Constant4/1 -> Sum18/1
  Sum35/1 -> kdroop/1
  Product3/1 -> Sum3/1
  Gain5/1 -> Low-Pass Filter (Discrete or Continuous)2/1
  iqs/1 -> Product3/2
  Pref/1 -> Sum35/1
  Sum18/1 -> Integrator2/1
  Low-Pass Filter (Discrete or Continuous)2/1 -> Scope4/1, Sum35/2
  Sum3/1 -> Gain5/1  "V_0_s"
  ids/1 -> Product5/2
  Product5/1 -> Sum3/2

== system myLibrary/AC-GFOR_DC-GFOL/Control Pac2/Rotació ==
  V_q_diff : Inport
  V_d_diff : Inport  Port=2
  V_0_diff : Inport  Port=3
  Angle : Inport  Port=4
  Constant{2,5..7} (4 alike) : Constant  Value=0
  Constant8 : Constant
  Demux : Demux  Outputs=3
  Display : Display
  Gain1 : Gain  Gain=-1
  Matrix Concatenate : Concatenate  NumInputs=3  Mode=Multidimensional array  ConcatenateDimension=2
  Mux{,1..3} (4 alike) : Mux  Inputs=3
  Product : Product  Multiplication=Matrix(*)
  Trigonometric Function : Trigonometry  Operator=cos
  Trigonometric Function1 : Trigonometry
  Trigonometric Function2 : Trigonometry
  Trigonometric Function3 : Trigonometry  Operator=cos
  V_alfa_diff : Outport  VectorParamsAs1DForOutWhenUnconnected=off
  V_beta_diff : Outport  Port=2  VectorParamsAs1DForOutWhenUnconnected=off
  V_0 : Outport  Port=3  VectorParamsAs1DForOutWhenUnconnected=off
  wires:
  Angle/1 -> Trigonometric Function1/1, Trigonometric Function2/1, Trigonometric Function3/1, Trigonometric Function/1
  Trigonometric Function2/1 -> Mux2/1
  Gain1/1 -> Mux1/2
  Trigonometric Function/1 -> Mux1/1
  V_0_diff/1 -> Mux/3
  V_d_diff/1 -> Mux/2
  V_q_diff/1 -> Mux/1
  Matrix Concatenate/1 -> Product/1, Display/1
  Mux/1 -> Product/2
  Demux/3 -> V_0/1
  Demux/2 -> V_beta_diff/1
  Demux/1 -> V_alfa_diff/1
  Product/1 -> Demux/1
  Mux1/1 -> Matrix Concatenate/1
  Mux3/1 -> Matrix Concatenate/3
  Mux2/1 -> Matrix Concatenate/2
  Constant8/1 -> Mux3/3
  Constant7/1 -> Mux3/2
  Constant6/1 -> Mux3/1
  Constant5/1 -> Mux2/3
  Trigonometric Function3/1 -> Mux2/2
  Constant2/1 -> Mux1/3
  Trigonometric Function1/1 -> Gain1/1

== system myLibrary/AC-GFOR_DC-GFOL/Control Pac2/Subsystem4 ==
  vq_ref : Inport
  vd_ref : Inport  Port=2
  vq : Inport  Port=3
  vd : Inport  Port=4
  Constant : Constant  Value=2*pi*T_IPC.fb
  Display1 : Display
  Display5 : Display
  Gain : Gain  Gain=T_IPC.Cac
  Integrator1 : Integrator  InitialCondition=initIPC.PI_vacq
  Integrator2 : Integrator  InitialCondition=initIPC.PI_vacd
  Product3 : Product  RndMeth=Zero
  Product4 : Product  RndMeth=Zero
  Scope : Scope  NumInputPorts=2
  Scope1 : Scope  NumInputPorts=2
  Scope2 : Scope  NumInputPorts=2
  Sum1 : Sum  Inputs=|+-
  Sum10 : Sum  Inputs=|++
  Sum2 : Sum  Inputs=|++
  Sum3 : Sum  Inputs=-+|
  Sum5 : Sum  Inputs=-+|
  Sum8 : Sum  Inputs=|++
  k1 : Gain  Gain=T_IPC.kpVac
  k2 : Gain  Gain=T_IPC.kiVac
  k3 : Gain  Gain=T_IPC.kpVac
  k4 : Gain  Gain=T_IPC.kiVac
  vd1 : InportShadow  Port=4
  vq1 : InportShadow  Port=3
  iqref : Outport  VectorParamsAs1DForOutWhenUnconnected=off
  idref : Outport  Port=2  VectorParamsAs1DForOutWhenUnconnected=off
  wires:
  Product4/1 -> Sum2/2
  Gain/1 -> Product3/2, Product4/1
  Constant/1 -> Gain/1
  Product3/1 -> Sum5/1
  Sum2/1 -> iqref/1
  Integrator2/1 -> Scope2/2, Display1/1, Sum10/2
  Sum1/1 -> k3/1, k2/1
  k3/1 -> Sum8/1
  Sum10/1 -> Sum5/2
  Integrator1/1 -> Scope2/1, Sum8/2, Display5/1
  vq_ref/1 -> Scope/1, Sum1/1
  Sum5/1 -> idref/1
  vd_ref/1 -> Scope1/2, Sum3/2
  k2/1 -> Integrator1/1
  k1/1 -> Sum10/1
  Sum3/1 -> k1/1, k4/1
  k4/1 -> Integrator2/1
  vq/1 -> Scope/2, Sum1/2
  vd/1 -> Scope1/1, Sum3/1
  Sum8/1 -> Sum2/1
  vq1/1 -> Product3/1
  vd1/1 -> Product4/2

== system myLibrary/AC-GFOR_DC-GFOL/Control Pac2/l_DC_alfa//beta ==
  Iabc_sum : Inport
  Clarke : Subsystem
  Ialfa_sum : Outport  VectorParamsAs1DForOutWhenUnconnected=off
  Ibeta_sum : Outport  Port=2  VectorParamsAs1DForOutWhenUnconnected=off
  I0_sum : Outport  Port=3  VectorParamsAs1DForOutWhenUnconnected=off
  wires:
  Iabc_sum/1 -> Clarke/1(Isum)
  Clarke/3(I_0) -> I0_sum/1
  Clarke/2(I_beta) -> Ibeta_sum/1
  Clarke/1(I_alfa) -> Ialfa_sum/1

== system myLibrary/AC-GFOR_DC-GFOL/MMC1/Controlled Voltage Source2 ==
  s : Inport
  ControlledVoltageSource : PMComponent  PhysicalDomain=powersysdomain  LeftPortType=p1  RightPortType=p1  LConnTagsString=a  RConnTagsString=__new0  mask(InnerPowersysBlock){}
      mask Display: disp('SPS internal use\nDo not delete')
  - : PMIOPort  Side=Left
  + : PMIOPort  Port=2  Side=Right
  tag scope: LibraryTag=global
  wires:
  s/1 -> [LibraryTag]
  connections:
  ControlledVoltageSource/RConn1 -- +/RConn1
  -/RConn1 -- ControlledVoltageSource/LConn1

== system myLibrary/AC-GFOR_DC-GFOL/MMC1/Controlled Voltage Source3 ==
  s : Inport
  ControlledVoltageSource : PMComponent  PhysicalDomain=powersysdomain  LeftPortType=p1  RightPortType=p1  LConnTagsString=a  RConnTagsString=__new0  mask(InnerPowersysBlock){}
      mask Display: disp('SPS internal use\nDo not delete')
  - : PMIOPort  Side=Left
  + : PMIOPort  Port=2  Side=Right
  tag scope: LibraryTag=global
  wires:
  s/1 -> [LibraryTag]
  connections:
  -/RConn1 -- ControlledVoltageSource/LConn1
  ControlledVoltageSource/RConn1 -- +/RConn1

== system myLibrary/GFOL/Control/Active Power Control ==
  Pac_ref : Inport
  w : Inport  Port=2
  id : Inport  Port=3
  iq : Inport  Port=4
  Ud : Inport  Port=5
  Uq : Inport  Port=6
  Constant : Constant  Value=T_VSC.wb
  Gain : Gain  Gain=3/2
  Integrator : Integrator  InitialCondition=initVSC.idiffq
  Ki : Gain  Gain=T_VSC.ki_P
  Kp : Gain  Gain=T_VSC.kp_P
  Low-Pass Filter (Discrete or Continuous)4 : eeGeneralControl/Low-Pass Filter (Discrete or Continuous)  K=1  T=T_VSC.tau_droop_f  B=inf  A=-inf  init_option=Specify as parameter  x0=T_VSC.wb  Ts=-1
  Product1 : Product
  Product3 : Product
  Scope : Scope  NumInputPorts=2
  Sum : Sum  Inputs=+-+
  Sum1 : Sum
  Sum2 : Sum  Inputs=|+-
  Sum4 : Sum
  droop : Gain  Gain=T_VSC.k_droop_f/T_VSC.wb
  Iq_ref : Outport
  wires:
  droop/1 -> Sum/3
  w/1 -> Low-Pass Filter (Discrete or Continuous)4/1
  Constant/1 -> Sum2/1
  Sum2/1 -> droop/1
  Low-Pass Filter (Discrete or Continuous)4/1 -> Sum2/2
  Uq/1 -> Product3/1
  iq/1 -> Product3/2
  Ud/1 -> Product1/1
  id/1 -> Product1/2
  Product3/1 -> Sum1/1
  Product1/1 -> Sum1/2
  Sum1/1 -> Gain/1
  Pac_ref/1 -> Scope/1, Sum/1
  Gain/1 -> Scope/2, Sum/2
  Integrator/1 -> Sum4/1
  Kp/1 -> Sum4/2
  Ki/1 -> Integrator/1
  Sum/1 -> Ki/1, Kp/1
  Sum4/1 -> Iq_ref/1

== system myLibrary/GFOL/Control/Clarke Anti-Transformation ==
  V_alfa_diff : Inport
  V_beta_dfff : Inport  Port=2
  V_0_diff : Inport  Port=3
  Constant{,2,5,8} (4 alike) : Constant
  Constant1 : Constant  Value=0
  Constant3 : Constant  Value=-1/2
  Constant4 : Constant  Value=-sqrt(3)/2
  Constant6 : Constant  Value=-1/2
  Constant7 : Constant  Value=sqrt(3)/2
  Demux : Demux  Outputs=3
  Display : Display
  Math Function : Math  Operator=transpose  SignedPower=on
  Matrix Concatenate : Concatenate  NumInputs=3  Mode=Multidimensional array  ConcatenateDimension=2
  Mux{,1..3} (4 alike) : Mux  Inputs=3
  Product : Product  Multiplication=Matrix(*)
  Va_diff : Outport  VectorParamsAs1DForOutWhenUnconnected=off
  Vb_diff : Outport  Port=2  VectorParamsAs1DForOutWhenUnconnected=off
  Vc_diff : Outport  Port=3  VectorParamsAs1DForOutWhenUnconnected=off
  wires:
  Constant/1 -> Mux1/1
  Constant1/1 -> Mux1/2
  Constant2/1 -> Mux1/3
  Constant3/1 -> Mux2/1
  Constant4/1 -> Mux2/2
  Constant5/1 -> Mux2/3
  Constant6/1 -> Mux3/1
  Constant7/1 -> Mux3/2
  Constant8/1 -> Mux3/3
  Matrix Concatenate/1 -> Math Function/1
  Mux2/1 -> Matrix Concatenate/2
  Mux3/1 -> Matrix Concatenate/3
  Mux1/1 -> Matrix Concatenate/1
  Product/1 -> Demux/1
  Demux/1 -> Va_diff/1  "Va"
  Demux/2 -> Vb_diff/1  "Vb"
  Demux/3 -> Vc_diff/1  "Vc"
  Mux/1 -> Product/2
  Math Function/1 -> Display/1, Product/1
  V_alfa_diff/1 -> Mux/1  "Valfa"
  V_beta_dfff/1 -> Mux/2  "Vbeta"
  V_0_diff/1 -> Mux/3  "0"

== system myLibrary/GFOL/Control/Conditional unit delay ==
  In1 : Inport
  Constant4 : Constant  Value=T_VSC.tau_cmd
  Switch : Switch  Criteria=u2 > Threshold  SaturateOnIntegerOverflow=off  InputSameDT=off
  Unit Delay2 : UnitDelay  InitialCondition=initVSC.vdiffq  SampleTime=T_VSC.tau_cmd  HasFrameUpgradeWarning=on
  Out1 : Outport
  wires:
  Constant4/1 -> Switch/2
  In1/1 -> Unit Delay2/1, Switch/3
  Unit Delay2/1 -> Switch/1
  Switch/1 -> Out1/1

== system myLibrary/GFOL/Control/Conditional zoh ==
  In1 : Inport
  Constant4 : Constant  Value=T_VSC.tau_zoh
  Switch : Switch  Criteria=u2 > Threshold  SaturateOnIntegerOverflow=off  InputSameDT=off
  Zero-Order Hold9 : ZeroOrderHold  SampleTime=T_VSC.tau_zoh
  Out1 : Outport
  wires:
  In1/1 -> Zero-Order Hold9/1, Switch/3
  Zero-Order Hold9/1 -> Switch/1
  Constant4/1 -> Switch/2
  Switch/1 -> Out1/1

== system myLibrary/GFOL/Control/Current Control ==
  Iq* : Inport
  Iq : Inport  Port=2
  Id* : Inport  Port=3
  Id : Inport  Port=4
  uq : Inport  Port=5
  ud : Inport  Port=6
  Constant : Constant  Value=T_VSC.wb
  Id1 : InportShadow  Port=4
  Integrator : Integrator  InitialCondition=initVSC.PI_idiffq
  Integrator1 : Integrator  InitialCondition=initVSC.PI_idiffd
  Iq1 : InportShadow  Port=2
  Ki : Gain  Gain=T_VSC.ki_s
  Ki1 : Gain  Gain=T_VSC.ki_s
  Kp : Gain  Gain=T_VSC.kp_s
  Kp1 : Gain  Gain=T_VSC.kp_s
  Lc : Gain  Gain=T_VSC.Lc
  Product : Product
  Product1 : Product
  Scope : Scope  NumInputPorts=2
  Sum : Sum  Inputs=|+-
  Sum1 : Sum  Inputs=|+-
  Sum2 : Sum  Inputs=+++
  Sum3 : Sum  Inputs=-++
  Sum4 : Sum
  Sum5 : Sum
  V_q_s : Outport  VectorParamsAs1DForOutWhenUnconnected=off
  V_d_s : Outport  Port=2  VectorParamsAs1DForOutWhenUnconnected=off
  wires:
  Sum2/1 -> V_q_s/1
  Sum5/1 -> Sum3/2
  Kp1/1 -> Sum5/2
  Integrator1/1 -> Sum5/1
  Ki1/1 -> Integrator1/1
  Sum1/1 -> Ki1/1, Kp1/1  "Error"
  Kp/1 -> Sum4/2
  Ki/1 -> Integrator/1
  Sum/1 -> Kp/1, Ki/1
  Lc/1 -> Product/2, Product1/1
  Id/1 -> Scope/2, Sum1/2
  Iq/1 -> Sum/2
  Iq*/1 -> Sum/1
  Constant/1 -> Lc/1
  ud/1 -> Sum3/3
  Sum4/1 -> Sum2/1
  uq/1 -> Sum2/3
  Sum3/1 -> V_d_s/1
  Product/1 -> Sum3/1
  Product1/1 -> Sum2/2
  Iq1/1 -> Product/1
  Id1/1 -> Product1/2
  Integrator/1 -> Sum4/1
  Id*/1 -> Scope/1, Sum1/1

== system myLibrary/GFOL/Control/Is ==
  Ias : Inport
  Ibs : Inport  Port=2
  Ics : Inport  Port=3
  Angle : Inport  Port=4
  Demux1 : Demux  Outputs=3
  Matriu T : Subsystem
  Mux : Mux  Inputs=3
  Product : Product  Multiplication=Matrix(*)
  Terminator : Terminator
  I_q_s : Outport  VectorParamsAs1DForOutWhenUnconnected=off
  I_d_s : Outport  Port=2  VectorParamsAs1DForOutWhenUnconnected=off
  wires:
  Product/1 -> Demux1/1
  Matriu T/1(Out1) -> Product/1
  Demux1/1 -> I_q_s/1
  Demux1/2 -> I_d_s/1
  Demux1/3 -> Terminator/1
  Angle/1 -> Matriu T/1(u)
  Mux/1 -> Product/2
  Ias/1 -> Mux/1
  Ibs/1 -> Mux/2
  Ics/1 -> Mux/3

== system myLibrary/GFOL/Control/Is1 ==
  Ias : Inport
  Ibs : Inport  Port=2
  Ics : Inport  Port=3
  Angle : Inport  Port=4
  Demux1 : Demux  Outputs=3
  Matriu T : Subsystem
  Mux : Mux  Inputs=3
  Product : Product  Multiplication=Matrix(*)
  I_q_s : Outport  VectorParamsAs1DForOutWhenUnconnected=off
  I_d_s : Outport  Port=2  VectorParamsAs1DForOutWhenUnconnected=off
  I_0_s : Outport  Port=3  VectorParamsAs1DForOutWhenUnconnected=off
  wires:
  Ics/1 -> Mux/3
  Ibs/1 -> Mux/2
  Ias/1 -> Mux/1
  Mux/1 -> Product/2
  Angle/1 -> Matriu T/1(u)
  Demux1/3 -> I_0_s/1
  Demux1/2 -> I_d_s/1
  Demux1/1 -> I_q_s/1
  Matriu T/1(Out1) -> Product/1
  Product/1 -> Demux1/1

== system myLibrary/GFOL/Control/Is3 ==
  Ias : Inport
  Ibs : Inport  Port=2
  Ics : Inport  Port=3
  Angle : Inport  Port=4
  Demux1 : Demux  Outputs=3
  Matriu T : Subsystem
  Mux : Mux  Inputs=3
  Product : Product  Multiplication=Matrix(*)
  I_q_s : Outport  VectorParamsAs1DForOutWhenUnconnected=off
  I_d_s : Outport  Port=2  VectorParamsAs1DForOutWhenUnconnected=off
  I_0_s : Outport  Port=3  VectorParamsAs1DForOutWhenUnconnected=off
  wires:
  Product/1 -> Demux1/1
  Matriu T/1(Out1) -> Product/1
  Demux1/1 -> I_q_s/1
  Demux1/2 -> I_d_s/1
  Demux1/3 -> I_0_s/1
  Angle/1 -> Matriu T/1(u)
  Mux/1 -> Product/2
  Ias/1 -> Mux/1
  Ibs/1 -> Mux/2
  Ics/1 -> Mux/3

== system myLibrary/GFOL/Control/Is4 ==
  Ias : Inport
  Ibs : Inport  Port=2
  Ics : Inport  Port=3
  Angle : Inport  Port=4
  Demux1 : Demux  Outputs=3
  Matriu T : Subsystem
  Mux : Mux  Inputs=3
  Product : Product  Multiplication=Matrix(*)
  I_q_s : Outport  VectorParamsAs1DForOutWhenUnconnected=off
  I_d_s : Outport  Port=2  VectorParamsAs1DForOutWhenUnconnected=off
  I_0_s : Outport  Port=3  VectorParamsAs1DForOutWhenUnconnected=off
  wires:
  Ics/1 -> Mux/3
  Ibs/1 -> Mux/2
  Ias/1 -> Mux/1
  Mux/1 -> Product/2
  Angle/1 -> Matriu T/1(u)
  Demux1/3 -> I_0_s/1
  Demux1/2 -> I_d_s/1
  Demux1/1 -> I_q_s/1
  Matriu T/1(Out1) -> Product/1
  Product/1 -> Demux1/1

== system myLibrary/GFOL/Control/Is5 ==
  Ias : Inport
  Ibs : Inport  Port=2
  Ics : Inport  Port=3
  Angle : Inport  Port=4
  Demux1 : Demux  Outputs=3
  Matriu T : Subsystem
  Mux : Mux  Inputs=3
  Product : Product  Multiplication=Matrix(*)
  I_q_s : Outport  VectorParamsAs1DForOutWhenUnconnected=off
  I_d_s : Outport  Port=2  VectorParamsAs1DForOutWhenUnconnected=off
  I_0_s : Outport  Port=3  VectorParamsAs1DForOutWhenUnconnected=off
  wires:
  Product/1 -> Demux1/1
  Matriu T/1(Out1) -> Product/1
  Demux1/1 -> I_q_s/1
  Demux1/2 -> I_d_s/1
  Demux1/3 -> I_0_s/1
  Angle/1 -> Matriu T/1(u)
  Mux/1 -> Product/2
  Ias/1 -> Mux/1
  Ibs/1 -> Mux/2
  Ics/1 -> Mux/3

== system myLibrary/GFOL/Control/Is7 ==
  Ias : Inport
  Ibs : Inport  Port=2
  Ics : Inport  Port=3
  Angle : Inport  Port=4
  Demux1 : Demux  Outputs=3
  Matriu T : Subsystem
  Mux : Mux  Inputs=3
  Product : Product  Multiplication=Matrix(*)
  I_q_s : Outport  VectorParamsAs1DForOutWhenUnconnected=off
  I_d_s : Outport  Port=2  VectorParamsAs1DForOutWhenUnconnected=off
  I_0_s : Outport  Port=3  VectorParamsAs1DForOutWhenUnconnected=off
  wires:
  Ics/1 -> Mux/3
  Ibs/1 -> Mux/2
  Ias/1 -> Mux/1
  Mux/1 -> Product/2
  Angle/1 -> Matriu T/1(u)
  Demux1/3 -> I_0_s/1
  Demux1/2 -> I_d_s/1
  Demux1/1 -> I_q_s/1
  Matriu T/1(Out1) -> Product/1
  Product/1 -> Demux1/1

== system myLibrary/GFOL/Control/PLL ==
  note: PLL
  U : Inport
  Ud : Inport  Port=2
  Constant : Constant  Value=0
  Constant1 : Constant
  Demux : Demux  Outputs=3
  Integrator : Integrator  InitialCondition=initVSC.thetaPLL_init
  Integrator1 : Integrator
  Ki : Gain  Gain=T_VSC.ki_pll
  Kp : Gain  Gain=T_VSC.kp_pll
  Scope1 : Scope
  Scope4 : Scope  NumInputPorts=2
  Sum : Sum  Inputs=|+-
  Sum1 : Sum  Inputs=|++
  Sum2 : Sum  Inputs=|++
  Terminator : Terminator
  Tpark : Subsystem
  wb : Gain  Gain=T_VSC.wb
  Angle : Outport
  Vzq : Outport  Port=2
  Vzd : Outport  Port=3
  w : Outport  Port=4
  wires:
  wb/1 -> Integrator/1, w/1
  Sum2/1 -> Scope1/1, wb/1
  Tpark/2(Vd) -> Vzd/1
  Constant1/1 -> Sum2/2
  Sum1/1 -> Sum2/1
  Tpark/3(0) -> Terminator/1
  Integrator/1 -> Angle/1, Tpark/4(u)
  Integrator1/1 -> Sum1/2
  Kp/1 -> Sum1/1
  Ki/1 -> Integrator1/1
  Sum/1 -> Kp/1, Ki/1
  Constant/1 -> Scope4/1, Sum/1
  Demux/1 -> Tpark/1(Va)
  Demux/3 -> Tpark/3(Vc)
  Demux/2 -> Tpark/2(Vb)
  U/1 -> Demux/1
  Tpark/1(Vq) -> Vzq/1
  Ud/1 -> Scope4/2, Sum/2

== system myLibrary/GFOL/Control/Reactive Power Control ==
  Q_ref : Inport
  id : Inport  Port=2
  iq : Inport  Port=3
  Ud : Inport  Port=4
  Uq : Inport  Port=5
  Gain : Gain  Gain=3/2
  Integrator : Integrator  InitialCondition=initVSC.idiffd
  Ki : Gain  Gain=T_VSC.ki_Q
  Kp : Gain  Gain=T_VSC.kp_Q
  Product1 : Product
  Product3 : Product
  Scope : Scope  NumInputPorts=2
  Sum : Sum  Inputs=|+-
  Sum1 : Sum  Inputs=+-
  Sum4 : Sum
  Id_ref : Outport
  wires:
  Sum4/1 -> Id_ref/1
  Sum/1 -> Kp/1, Ki/1
  Ki/1 -> Integrator/1
  Kp/1 -> Sum4/2
  Integrator/1 -> Sum4/1
  Q_ref/1 -> Scope/1, Sum/1
  Sum1/1 -> Gain/1
  Product1/1 -> Sum1/2
  Product3/1 -> Sum1/1
  Ud/1 -> Product1/1
  Uq/1 -> Product3/1
  id/1 -> Product3/2
  iq/1 -> Product1/2
  Gain/1 -> Scope/2, Sum/2
